simulink model "Formation_demo_app1"  (R2019a)
settings: Solver=VariableStepAuto  StartTime=0.0  StopTime=180  RelTol=1e-3
values from neighbouring files (symbols this model uses):
  K1 = [-2, -1.2]    [Application1.m]
  K2 = [0.3416, 0.7330]    [Application1.m]
  r = 7    [Application1.m]
  Theta_ini = [Theta_ini_1, Theta_ini_2, Theta_ini_3, Theta_ini_4, Theta_ini_5]'    [Application1.m]
  w = 0.214    [Application1.m]
settings Model: Creator=kocab  LastModifiedBy=Kocab

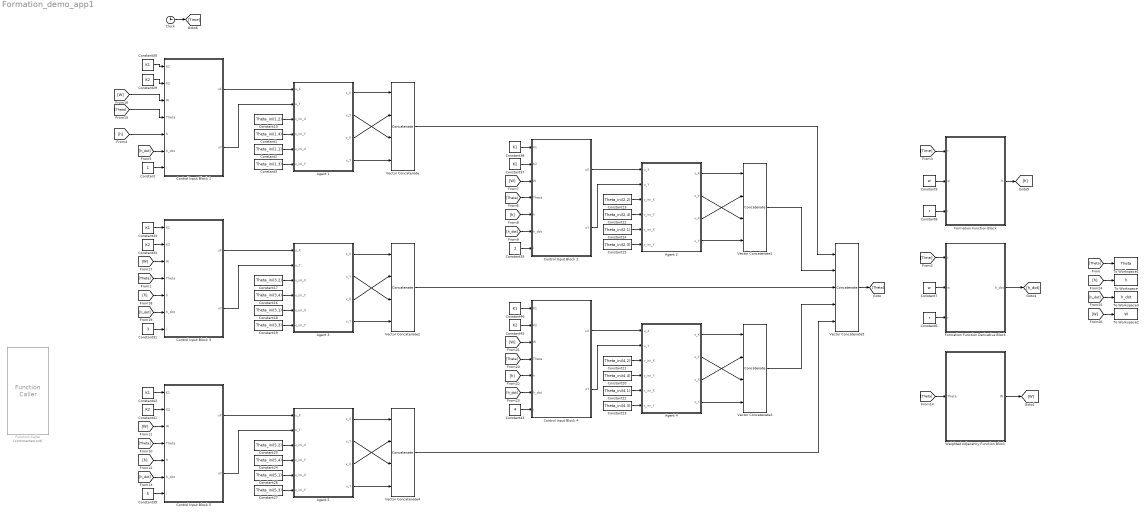
== system Formation_demo_app1 ==
  Agent 1 : Subsystem
  Agent 2 : Subsystem
  Agent 3 : Subsystem
  Agent 4 : Subsystem
  Agent 5 : Subsystem
  Clock : Clock
  Constant : Constant
  Constant1 : Constant  Value=Theta_ini(1,4)
  Constant10 : Constant  Value=Theta_ini(1,2)
  Constant12 : Constant  Value=Theta_ini(2,4)
  Constant13 : Constant  Value=Theta_ini(2,2)
  Constant14 : Constant  Value=Theta_ini(2,1)
  Constant15 : Constant  Value=Theta_ini(2,3)
  Constant16 : Constant  Value=Theta_ini(3,4)
  Constant17 : Constant  Value=Theta_ini(3,2)
  Constant18 : Constant  Value=Theta_ini(3,1)
  Constant19 : Constant  Value=Theta_ini(3,3)
  Constant2 : Constant  Value=Theta_ini(1,1)
  Constant20 : Constant  Value=Theta_ini(4,4)
  Constant21 : Constant  Value=Theta_ini(4,2)
  Constant22 : Constant  Value=Theta_ini(4,1)
  Constant23 : Constant  Value=Theta_ini(4,3)
  Constant24 : Constant  Value=Theta_ini(5,4)
  Constant25 : Constant  Value=Theta_ini(5,2)
  Constant26 : Constant  Value=Theta_ini(5,1)
  Constant27 : Constant  Value=Theta_ini(5,3)
  Constant{29,33,37,41,45} (5 alike) : Constant  Value=K2
  Constant3 : Constant  Value=Theta_ini(1,3)
  Constant{30,34,38,42,46} (5 alike) : Constant  Value=K1
  Constant31 : Constant  Value=3
  Constant35 : Constant  Value=2
  Constant39 : Constant  Value=5
  Constant43 : Constant  Value=4
  Constant6 : Constant  Value=r
  Constant7 : Constant  Value=w
  Constant8 : Constant  Value=r
  Constant9 : Constant  Value=w
  Control Input Block 1 : MATLAB Function  TreatAsAtomicUnit=on
  Control Input Block 2 : MATLAB Function  TreatAsAtomicUnit=on
  Control Input Block 3 : MATLAB Function  TreatAsAtomicUnit=on
  Control Input Block 4 : MATLAB Function  TreatAsAtomicUnit=on
  Control Input Block 5 : MATLAB Function  TreatAsAtomicUnit=on
  Formation Function Block : MATLAB Function  TreatAsAtomicUnit=on
  Formation Function Derivative Block : MATLAB Function  TreatAsAtomicUnit=on
  Function Caller : FunctionCaller  Commented=on  FunctionPrototype=[uX,uY] = control_input(K1,K2,W,Theta,h,h_dot,i,num_agents)  InputArgumentSpecifications=<Enter example>  OutputArgumentSpecifications=<Enter example>
  To Workspace : ToWorkspace  VariableName=h  SaveFormat=Timeseries  SampleTime=-1
  To Workspace1 : ToWorkspace  VariableName=Theta  SaveFormat=Timeseries  SampleTime=-1
  To Workspace2 : ToWorkspace  VariableName=W  SaveFormat=Timeseries  SampleTime=-1
  To Workspace3 : ToWorkspace  VariableName=h_dot  SaveFormat=Timeseries  SampleTime=-1
  Vector Concatenate{,1..4} (5 alike) : Concatenate  NumInputs=4  Mode=Multidimensional array  ConcatenateDimension=2
  Vector Concatenate5 : Concatenate  NumInputs=5  Mode=Multidimensional array
  Weighted Adjacency Function Block : MATLAB Function  TreatAsAtomicUnit=on
  wires:
  Control Input Block 1/2(uY) -> Agent 1/2(u_Y)
  Constant2/1 -> Agent 1/5(x_ini_X)
  Constant3/1 -> Agent 1/6(x_ini_Y)
  Agent 1/2(x_Y) -> Vector Concatenate/3
  Constant10/1 -> Agent 1/3(v_ini_X)
  Agent 1/4(v_Y) -> Vector Concatenate/4
  Constant1/1 -> Agent 1/4(v_ini_Y)
  Agent 1/3(v_X) -> Vector Concatenate/2
  Agent 1/1(x_X) -> Vector Concatenate/1
  Control Input Block 1/1(uX) -> Agent 1/1(u_X)
  Formation Function Derivative Block/1(h_dot) -> [h_dot]
  Formation Function Block/1(h) -> [h]
  Constant7/1 -> Formation Function Derivative Block/2(w)
  Constant6/1 -> Formation Function Derivative Block/3(r)
  Constant9/1 -> Formation Function Block/2(w)
  Constant8/1 -> Formation Function Block/3(r)
  Clock/1 -> [Time]
  [Time] -> Formation Function Derivative Block/1(t)
  [Time] -> Formation Function Block/1(t)
  [h] -> Control Input Block 1/5(h)
  [h_dot] -> Control Input Block 1/6(h_dot)
  Constant/1 -> Control Input Block 1/7(i)
  Agent 2/1(x_X) -> Vector Concatenate1/1
  Constant14/1 -> Agent 2/5(x_ini_X)
  Agent 2/3(v_X) -> Vector Concatenate1/2
  Control Input Block 2/1(uX) -> Agent 2/1(u_X)
  Control Input Block 2/2(uY) -> Agent 2/2(u_Y)
  Constant15/1 -> Agent 2/6(x_ini_Y)
  Constant13/1 -> Agent 2/3(v_ini_X)
  Agent 2/2(x_Y) -> Vector Concatenate1/3
  Agent 2/4(v_Y) -> Vector Concatenate1/4
  Constant12/1 -> Agent 2/4(v_ini_Y)
  Agent 3/1(x_X) -> Vector Concatenate2/1
  Constant18/1 -> Agent 3/5(x_ini_X)
  Agent 3/3(v_X) -> Vector Concatenate2/2
  Control Input Block 3/1(uX) -> Agent 3/1(u_X)
  Control Input Block 3/2(uY) -> Agent 3/2(u_Y)
  Constant19/1 -> Agent 3/6(x_ini_Y)
  Constant17/1 -> Agent 3/3(v_ini_X)
  Agent 3/2(x_Y) -> Vector Concatenate2/3
  Agent 3/4(v_Y) -> Vector Concatenate2/4
  Constant16/1 -> Agent 3/4(v_ini_Y)
  Agent 4/1(x_X) -> Vector Concatenate3/1
  Constant22/1 -> Agent 4/5(x_ini_X)
  Agent 4/3(v_X) -> Vector Concatenate3/2
  Control Input Block 4/1(uX) -> Agent 4/1(u_X)
  Control Input Block 4/2(uY) -> Agent 4/2(u_Y)
  Constant23/1 -> Agent 4/6(x_ini_Y)
  Constant21/1 -> Agent 4/3(v_ini_X)
  Agent 4/2(x_Y) -> Vector Concatenate3/3
  Agent 4/4(v_Y) -> Vector Concatenate3/4
  Constant20/1 -> Agent 4/4(v_ini_Y)
  Agent 5/1(x_X) -> Vector Concatenate4/1
  Constant26/1 -> Agent 5/5(x_ini_X)
  Agent 5/3(v_X) -> Vector Concatenate4/2
  Control Input Block 5/1(uX) -> Agent 5/1(u_X)
  Control Input Block 5/2(uY) -> Agent 5/2(u_Y)
  Constant27/1 -> Agent 5/6(x_ini_Y)
  Constant25/1 -> Agent 5/3(v_ini_X)
  Agent 5/2(x_Y) -> Vector Concatenate4/3
  Agent 5/4(v_Y) -> Vector Concatenate4/4
  Constant24/1 -> Agent 5/4(v_ini_Y)
  Vector Concatenate4/1 -> Vector Concatenate5/5
  Vector Concatenate3/1 -> Vector Concatenate5/4
  Vector Concatenate2/1 -> Vector Concatenate5/3
  Vector Concatenate1/1 -> Vector Concatenate5/2
  Vector Concatenate/1 -> Vector Concatenate5/1
  Vector Concatenate5/1 -> [Theta]
  [Theta] -> Weighted Adjacency Function Block/1(Theta)
  Weighted Adjacency Function Block/1(W) -> [W]
  [Theta] -> Control Input Block 1/4(Theta)
  [W] -> Control Input Block 1/3(W)
  Constant29/1 -> Control Input Block 1/2(K2)
  Constant30/1 -> Control Input Block 1/1(K1)
  [h] -> Control Input Block 3/5(h)
  Constant34/1 -> Control Input Block 3/1(K1)
  [h_dot] -> Control Input Block 3/6(h_dot)
  Constant33/1 -> Control Input Block 3/2(K2)
  [Theta] -> Control Input Block 3/4(Theta)
  Constant31/1 -> Control Input Block 3/7(i)
  [W] -> Control Input Block 3/3(W)
  [h] -> Control Input Block 2/5(h)
  Constant38/1 -> Control Input Block 2/1(K1)
  [h_dot] -> Control Input Block 2/6(h_dot)
  Constant37/1 -> Control Input Block 2/2(K2)
  [Theta] -> Control Input Block 2/4(Theta)
  Constant35/1 -> Control Input Block 2/7(i)
  [W] -> Control Input Block 2/3(W)
  [h] -> Control Input Block 5/5(h)
  Constant42/1 -> Control Input Block 5/1(K1)
  [h_dot] -> Control Input Block 5/6(h_dot)
  Constant41/1 -> Control Input Block 5/2(K2)
  [Theta] -> Control Input Block 5/4(Theta)
  Constant39/1 -> Control Input Block 5/7(i)
  [W] -> Control Input Block 5/3(W)
  [h] -> Control Input Block 4/5(h)
  Constant46/1 -> Control Input Block 4/1(K1)
  [h_dot] -> Control Input Block 4/6(h_dot)
  Constant45/1 -> Control Input Block 4/2(K2)
  [Theta] -> Control Input Block 4/4(Theta)
  Constant43/1 -> Control Input Block 4/7(i)
  [W] -> Control Input Block 4/3(W)
  [W] -> To Workspace2/1
  [h_dot] -> To Workspace3/1
  [h] -> To Workspace/1
  [Theta] -> To Workspace1/1

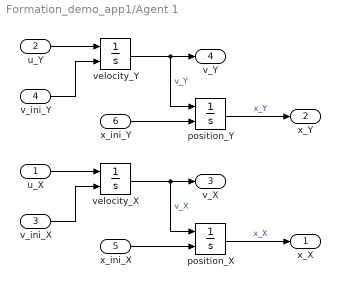
== system Formation_demo_app1/Agent 1 ==
  u_X : Inport
  u_Y : Inport  Port=2
  v_ini_X : Inport  Port=3
  v_ini_Y : Inport  Port=4
  x_ini_X : Inport  Port=5
  x_ini_Y : Inport  Port=6
  position_X : Integrator  InitialConditionSource=external
  position_Y : Integrator  InitialConditionSource=external
  velocity_X : Integrator  InitialConditionSource=external
  velocity_Y : Integrator  InitialConditionSource=external
  x_X : Outport
  x_Y : Outport  Port=2
  v_X : Outport  Port=3
  v_Y : Outport  Port=4
  wires:
  velocity_X/1 -> position_X/1, v_X/1  "v_X"
  position_X/1 -> x_X/1  "x_X"
  v_ini_Y/1 -> velocity_Y/2
  velocity_Y/1 -> position_Y/1, v_Y/1  "v_Y"
  x_ini_Y/1 -> position_Y/2
  v_ini_X/1 -> velocity_X/2
  x_ini_X/1 -> position_X/2
  position_Y/1 -> x_Y/1  "x_Y"
  u_X/1 -> velocity_X/1
  u_Y/1 -> velocity_Y/1

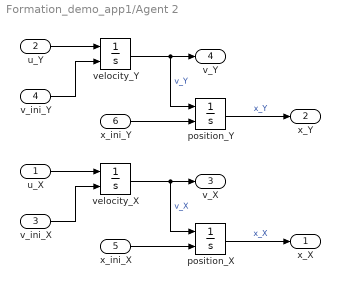
== system Formation_demo_app1/Agent 2 ==
  u_X : Inport
  u_Y : Inport  Port=2
  v_ini_X : Inport  Port=3
  v_ini_Y : Inport  Port=4
  x_ini_X : Inport  Port=5
  x_ini_Y : Inport  Port=6
  position_X : Integrator  InitialConditionSource=external
  position_Y : Integrator  InitialConditionSource=external
  velocity_X : Integrator  InitialConditionSource=external
  velocity_Y : Integrator  InitialConditionSource=external
  x_X : Outport
  x_Y : Outport  Port=2
  v_X : Outport  Port=3
  v_Y : Outport  Port=4
  wires:
  velocity_X/1 -> position_X/1, v_X/1  "v_X"
  position_X/1 -> x_X/1  "x_X"
  v_ini_Y/1 -> velocity_Y/2
  velocity_Y/1 -> position_Y/1, v_Y/1  "v_Y"
  x_ini_Y/1 -> position_Y/2
  v_ini_X/1 -> velocity_X/2
  x_ini_X/1 -> position_X/2
  position_Y/1 -> x_Y/1  "x_Y"
  u_X/1 -> velocity_X/1
  u_Y/1 -> velocity_Y/1

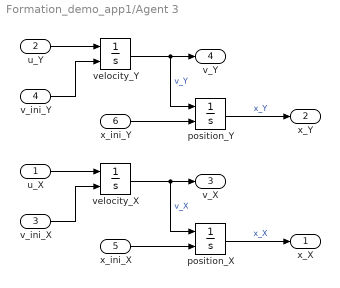
== system Formation_demo_app1/Agent 3 ==
  u_X : Inport
  u_Y : Inport  Port=2
  v_ini_X : Inport  Port=3
  v_ini_Y : Inport  Port=4
  x_ini_X : Inport  Port=5
  x_ini_Y : Inport  Port=6
  position_X : Integrator  InitialConditionSource=external
  position_Y : Integrator  InitialConditionSource=external
  velocity_X : Integrator  InitialConditionSource=external
  velocity_Y : Integrator  InitialConditionSource=external
  x_X : Outport
  x_Y : Outport  Port=2
  v_X : Outport  Port=3
  v_Y : Outport  Port=4
  wires:
  velocity_X/1 -> position_X/1, v_X/1  "v_X"
  position_X/1 -> x_X/1  "x_X"
  v_ini_Y/1 -> velocity_Y/2
  velocity_Y/1 -> position_Y/1, v_Y/1  "v_Y"
  x_ini_Y/1 -> position_Y/2
  v_ini_X/1 -> velocity_X/2
  x_ini_X/1 -> position_X/2
  position_Y/1 -> x_Y/1  "x_Y"
  u_X/1 -> velocity_X/1
  u_Y/1 -> velocity_Y/1

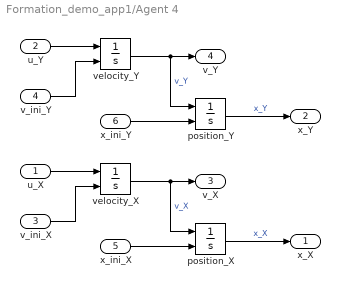
== system Formation_demo_app1/Agent 4 ==
  u_X : Inport
  u_Y : Inport  Port=2
  v_ini_X : Inport  Port=3
  v_ini_Y : Inport  Port=4
  x_ini_X : Inport  Port=5
  x_ini_Y : Inport  Port=6
  position_X : Integrator  InitialConditionSource=external
  position_Y : Integrator  InitialConditionSource=external
  velocity_X : Integrator  InitialConditionSource=external
  velocity_Y : Integrator  InitialConditionSource=external
  x_X : Outport
  x_Y : Outport  Port=2
  v_X : Outport  Port=3
  v_Y : Outport  Port=4
  wires:
  velocity_X/1 -> position_X/1, v_X/1  "v_X"
  position_X/1 -> x_X/1  "x_X"
  v_ini_Y/1 -> velocity_Y/2
  velocity_Y/1 -> position_Y/1, v_Y/1  "v_Y"
  x_ini_Y/1 -> position_Y/2
  v_ini_X/1 -> velocity_X/2
  x_ini_X/1 -> position_X/2
  position_Y/1 -> x_Y/1  "x_Y"
  u_X/1 -> velocity_X/1
  u_Y/1 -> velocity_Y/1

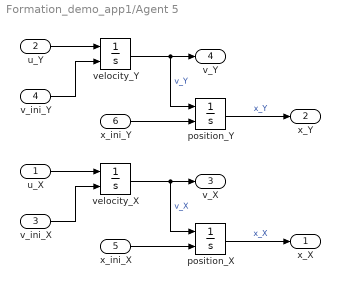
== system Formation_demo_app1/Agent 5 ==
  u_X : Inport
  u_Y : Inport  Port=2
  v_ini_X : Inport  Port=3
  v_ini_Y : Inport  Port=4
  x_ini_X : Inport  Port=5
  x_ini_Y : Inport  Port=6
  position_X : Integrator  InitialConditionSource=external
  position_Y : Integrator  InitialConditionSource=external
  velocity_X : Integrator  InitialConditionSource=external
  velocity_Y : Integrator  InitialConditionSource=external
  x_X : Outport
  x_Y : Outport  Port=2
  v_X : Outport  Port=3
  v_Y : Outport  Port=4
  wires:
  velocity_X/1 -> position_X/1, v_X/1  "v_X"
  position_X/1 -> x_X/1  "x_X"
  v_ini_Y/1 -> velocity_Y/2
  velocity_Y/1 -> position_Y/1, v_Y/1  "v_Y"
  x_ini_Y/1 -> position_Y/2
  v_ini_X/1 -> velocity_X/2
  x_ini_X/1 -> position_X/2
  position_Y/1 -> x_Y/1  "x_Y"
  u_X/1 -> velocity_X/1
  u_Y/1 -> velocity_Y/1

== matlab function Formation_demo_app1/Formation Function Derivative Block ==
  data: t input; w input; h_dot output size=[5 4] [-inf..inf]; r input
function h_dot = formation_func_dot(t, w, r)
    % Size: num_agents x 4 (i.e. 5 x 4)
    h_dot = zeros(5,4); % size: 5x4
    for i = 1:5
        h_dot(i,:)=[- w * r * sin(w*t + 2*pi*(i - 1)/5) * g_dummy(t,i,w), ...
                    - w^2 * r * cos(w*t + 2*pi*(i - 1)/5) * g_dummy(t,i,w),...
                    w * r * cos(w*t + 2*pi*(i - 1)/5),...
                    - w^2 * r * sin(w*t + 2*pi*(i - 1)/5)   ] ;
    end

== matlab function Formation_demo_app1/Formation Function Block ==
  data: t input; h output size=[5 4] [-inf..inf]; w input; r input
function h = formation_func(t, w, r)
    % Size: num_agents x 4 (i.e. 5 x 4)
    h = zeros(5,4); % size: 5x4
    for i = 1:5
        h(i,:)=[r * (cos((w*t) + 2*pi*(i-1)/5) - 1) * g_dummy(t,i,w), ...
                - w * r * sin(w*t + 2*pi*(i - 1)/5) * g_dummy(t,i,w),...
                r * sin(w*t + 2*pi*(i - 1)/5),...
                w * r * cos(w*t + 2*pi*(i - 1)/5)   ]' ;
    end
%     for i = 1:5
%         h(i,:)=[r * cos((w*t) + 2*pi*(i-1)/5 - 1), ...
%                 - w * r * sin(w*t + 2*pi*(i - 1)/5),...
%                 r * sin(w*t + 2*pi*(i - 1)/5 - 1),...
%                 w * r * cos(w*t + 2*pi*(i - 1)/5)   ]' ;
%     end

== matlab function Formation_demo_app1/Control Input Block 1 ==
  data: uX output; K1 input size=[1 2]; K2 input size=[1 2]; W input size=[5 5]; Theta input size=[5 4]; h input size=[5 4]; h_dot input size=[5 4]; i input; uY output
function [uX, uY] = control_input(K1, K2, W, Theta, h, h_dot, i)
    local_sum = zeros(4,1);  % size: 4x1
    for j = 1: 5
        local_sum = local_sum + ...
                    (W(i,j) * ( (Theta(j,:) - h(j,:)) ...
                                - (Theta(i,:)-h(i,:)) ...
                                )...
                    )' ; %% size 4x1
    end
    
    % size: 1st term: K1*Theta(i,X)         size: (1x2)*(2x1) = 1x1
    % size: 2nd term: K2*Summation(j-i,X)   size: (1x2)*(2x1) = 1x1
    % size: 3rd term: h_dot(i,Y)            size: (1x1)
    uX =    K1*(Theta(i,1:2)' - h(i,1:2)') ...
            + K2*local_sum(1:2,1) ...
            + h_dot(i,2) ;

    % size: 1st term: K1*Theta(i,Y)         size: (1x2)*(2x1) = 1x1
    % size: 2nd term: K2*Summation(j-i,Y)   size: (1x2)*(2x1) = 1x1
    % size: 3rd term: h_dot(i,Y)            size: (1x1)
    uY =    K1*(Theta(i,3:4)' - h(i,3:4)') ...
            + K2*local_sum(3:4 ,1) ...
            + h_dot(i,4) ;

== matlab function Formation_demo_app1/Weighted Adjacency Function Block ==
  data: W output size=[5 5] [-inf..inf]; Theta input size=[5 4]
function W = weighted_adjacency(Theta)
    W = zeros(5,5); % size: 5x5
%     for i = 1:5
%         for j = 1:5
%             if i == j
%                 W(i,j) = 0 ;
%             elseif i>j
%                 W(i,j) = norm( [Theta(i,1) - Theta(j,1) , Theta(i,3) - Theta(j,3)] ) ;
%             else
%                 W(i,j) = norm( [Theta(i,1) - Theta(j,1) , Theta(i,3) - Theta(j,3)] ) ;
%             end
%         end
%     end
%     for i = 1:5
%         for j = 1:5
%             if ( mod(i - 1 , 5) == mod(j,5) )
%                 W(i,j) = norm( [Theta(i,1) - Theta(j,1) , Theta(i,3) - Theta(j,3)] ) ;
%             elseif ( mod(i + 1 , 5) == mod(j,5) )
%                 W(i,j) = norm( [Theta(i,1) - Theta(j,1) , Theta(i,3) - Theta(j,3)] ) ;
%             end
%         end
%     end
    for i = 1:5
        for j = 1:5
            if ( mod(i - 1 , 5) == mod(j,5) )
                W(i,j) = 1 ;
            elseif ( mod(i + 1 , 5) == mod(j,5) )
                W(i,j) = 1 ;
            end
        end
    end

== matlab function Formation_demo_app1/Control Input Block 3 ==
  data: K1 input size=[1 2]; uX output; K2 input size=[1 2]; W input size=[5 5]; Theta input size=[5 4]; h input size=[5 4]; h_dot input size=[5 4]; i input; uY output
function [uX, uY] = control_input(K1, K2, W, Theta, h, h_dot, i)
    local_sum = zeros(4,1);  % size: 4x1
    for j = 1: 5
        local_sum = local_sum + ...
                    (W(i,j) * ( (Theta(j,:) - h(j,:)) ...
                                - (Theta(i,:)-h(i,:)) ...
                                )...
                    )' ; %% size 4x1
    end
    
    % size: 1st term: K1*Theta(i,X)         size: (1x2)*(2x1) = 1x1
    % size: 2nd term: K2*Summation(j-i,X)   size: (1x2)*(2x1) = 1x1
    % size: 3rd term: h_dot(i,Y)            size: (1x1)
    uX =    K1*(Theta(i,1:2)' - h(i,1:2)') ...
            + K2*local_sum(1:2,1) ...
            + h_dot(i,2) ;

    % size: 1st term: K1*Theta(i,Y)         size: (1x2)*(2x1) = 1x1
    % size: 2nd term: K2*Summation(j-i,Y)   size: (1x2)*(2x1) = 1x1
    % size: 3rd term: h_dot(i,Y)            size: (1x1)
    uY =    K1*(Theta(i,3:4)' - h(i,3:4)') ...
            + K2*local_sum(3:4 ,1) ...
            + h_dot(i,4) ;

== matlab function Formation_demo_app1/Control Input Block 2 ==
  data: K1 input size=[1 2]; uX output; K2 input size=[1 2]; W input size=[5 5]; Theta input size=[5 4]; h input size=[5 4]; h_dot input size=[5 4]; i input; uY output
function [uX, uY] = control_input(K1, K2, W, Theta, h, h_dot, i)
    local_sum = zeros(4,1);  % size: 4x1
    for j = 1: 5
        local_sum = local_sum + ...
                    (W(i,j) * ( (Theta(j,:) - h(j,:)) ...
                                - (Theta(i,:)-h(i,:)) ...
                                )...
                    )' ; %% size 4x1
    end
    
    % size: 1st term: K1*Theta(i,X)         size: (1x2)*(2x1) = 1x1
    % size: 2nd term: K2*Summation(j-i,X)   size: (1x2)*(2x1) = 1x1
    % size: 3rd term: h_dot(i,Y)            size: (1x1)
    uX =    K1*(Theta(i,1:2)' - h(i,1:2)') ...
            + K2*local_sum(1:2,1) ...
            + h_dot(i,2) ;

    % size: 1st term: K1*Theta(i,Y)         size: (1x2)*(2x1) = 1x1
    % size: 2nd term: K2*Summation(j-i,Y)   size: (1x2)*(2x1) = 1x1
    % size: 3rd term: h_dot(i,Y)            size: (1x1)
    uY =    K1*(Theta(i,3:4)' - h(i,3:4)') ...
            + K2*local_sum(3:4 ,1) ...
            + h_dot(i,4) ;

== matlab function Formation_demo_app1/Control Input Block 5 ==
  data: K1 input size=[1 2]; uX output; K2 input size=[1 2]; W input size=[5 5]; Theta input size=[5 4]; h input size=[5 4]; h_dot input size=[5 4]; i input; uY output
function [uX, uY] = control_input(K1, K2, W, Theta, h, h_dot, i)
    local_sum = zeros(4,1);  % size: 4x1
    for j = 1: 5
        local_sum = local_sum + ...
                    (W(i,j) * ( (Theta(j,:) - h(j,:)) ...
                                - (Theta(i,:)-h(i,:)) ...
                                )...
                    )' ; %% size 4x1
    end
    
    % size: 1st term: K1*Theta(i,X)         size: (1x2)*(2x1) = 1x1
    % size: 2nd term: K2*Summation(j-i,X)   size: (1x2)*(2x1) = 1x1
    % size: 3rd term: h_dot(i,Y)            size: (1x1)
    uX =    K1*(Theta(i,1:2)' - h(i,1:2)') ...
            + K2*local_sum(1:2,1) ...
            + h_dot(i,2) ;

    % size: 1st term: K1*Theta(i,Y)         size: (1x2)*(2x1) = 1x1
    % size: 2nd term: K2*Summation(j-i,Y)   size: (1x2)*(2x1) = 1x1
    % size: 3rd term: h_dot(i,Y)            size: (1x1)
    uY =    K1*(Theta(i,3:4)' - h(i,3:4)') ...
            + K2*local_sum(3:4 ,1) ...
            + h_dot(i,4) ;

== matlab function Formation_demo_app1/Control Input Block 4 ==
  data: K1 input size=[1 2]; uX output; K2 input size=[1 2]; W input size=[5 5]; Theta input size=[5 4]; h input size=[5 4]; h_dot input size=[5 4]; i input; uY output
function [uX, uY] = control_input(K1, K2, W, Theta, h, h_dot, i)
    local_sum = zeros(4,1);  % size: 4x1
    for j = 1: 5
        local_sum = local_sum + ...
                    (W(i,j) * ( (Theta(j,:) - h(j,:)) ...
                                - (Theta(i,:)-h(i,:)) ...
                                )...
                    )' ; %% size 4x1
    end
    
    % size: 1st term: K1*Theta(i,X)         size: (1x2)*(2x1) = 1x1
    % size: 2nd term: K2*Summation(j-i,X)   size: (1x2)*(2x1) = 1x1
    % size: 3rd term: h_dot(i,Y)            size: (1x1)
    uX =    K1*(Theta(i,1:2)' - h(i,1:2)') ...
            + K2*local_sum(1:2,1) ...
            + h_dot(i,2) ;

    % size: 1st term: K1*Theta(i,Y)         size: (1x2)*(2x1) = 1x1
    % size: 2nd term: K2*Summation(j-i,Y)   size: (1x2)*(2x1) = 1x1
    % size: 3rd term: h_dot(i,Y)            size: (1x1)
    uY =    K1*(Theta(i,3:4)' - h(i,3:4)') ...
            + K2*local_sum(3:4 ,1) ...
            + h_dot(i,4) ;
